simulink model "linear_model"  (Simulink 8.0)
settings: Solver=ode45  StartTime=0.0  StopTime=0.01  FixedStep=0.0001  RelTol=1e-3
settings Model: Creator=T-3000  LastModifiedBy=T-3000  BufferReuse=off
settings DataIOCC: SignalLoggingSaveFormat=ModelDataLogs  SignalLoggingName=sigsOut
settings OptimizationCC: InlineInvariantSignals=on  OptimizeBlockIOStorage=off  BufferReuse=off  ExpressionFolding=off  LocalBlockOutputs=off
settings DebuggingCC: SaveWithParameterizedLinksMsg=none  SignalResolutionControl=TryResolveAllWithWarning  SolverPrmCheckMsg=none  MultiTaskDSMMsg=warning  MultiTaskCondExecSysMsg=none  StrictBusMsg=None
settings HardwareCC: TargetUnknown=on
settings RTWCC: IncludeERTFirstTime=on
settings GRTTargetCC: CombineOutputUpdateFcns=off  GRTInterface=on

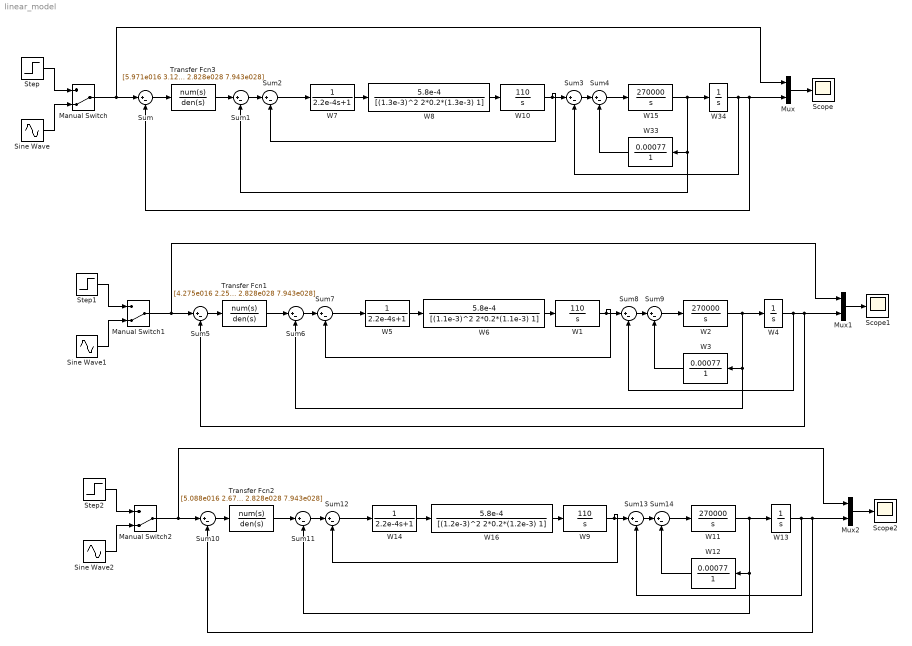
== system linear_model ==
  Manual Switch : ManualSwitch  CurrentSetting=0
  Manual Switch1 : ManualSwitch  CurrentSetting=0
  Manual Switch2 : ManualSwitch  CurrentSetting=0
  Mux : Mux  Inputs=2
  Mux1 : Mux  Inputs=2
  Mux2 : Mux  Inputs=2
  Scope : Scope
      settings: TimeRange=5  YMin=0  YMax=1.2
  Scope1 : Scope
      settings: TimeRange=5  YMin=0  YMax=1
  Scope2 : Scope
      settings: TimeRange=5  YMin=0  YMax=1  SaveName=ScopeData2
  Sine Wave : Sin  Frequency=1200  SampleTime=0
  Sine Wave1 : Sin  Frequency=1200  SampleTime=0
  Sine Wave2 : Sin  Frequency=1200  SampleTime=0
  Step : Step  Time=0  SampleTime=0
  Step1 : Step  Time=0  SampleTime=0
  Step2 : Step  Time=0  SampleTime=0
  Sum{,1..14} (15 alike) : Sum  Inputs=|+-  SaturateOnIntegerOverflow=on
  Transfer Fcn1 : TransferFcn  Numerator=[4.275e016 2.258e020 1.99e023 2.742e026 1.061e029 6.01e031 7.477e033 9.532e032]  Denominator=[1 1.539e006 8.565e011 2.152e017 2.439e022 1.001e027 2.828e028 7.943e028]
  Transfer Fcn2 : TransferFcn  Numerator=[5.088e016 2.672e020 2.225e023 2.902e026 1.101e029 6.04e031 7.477e033 9.532e032]  Denominator=[1 1.539e006 8.565e011 2.152e017 2.439e022 1.001e027 2.828e028 7.943e028]
  Transfer Fcn3 : TransferFcn  Numerator=[5.971e016 3.121e020 2.475e023 3.073e026 1.143e029 6.07e031 7.477e033 9.532e032]  Denominator=[1 1.539e006 8.565e011 2.152e017 2.439e022 1.001e027 2.828e028 7.943e028]
  W1 : TransferFcn  Numerator=[110]  Denominator=[1 0]
  W10 : TransferFcn  Numerator=[110]  Denominator=[1 0]
  W11 : TransferFcn  Numerator=[270000]  Denominator=[1 0]
  W12 : TransferFcn  Numerator=[0.00077]  Denominator=[1]
  W13 : TransferFcn  Denominator=[1 0]
  W14 : TransferFcn  Denominator=[2.2e-4 1]
  W15 : TransferFcn  Numerator=[270000]  Denominator=[1 0]
  W16 : TransferFcn  Numerator=[5.8e-4]  Denominator=[(1.2e-3)^2 2*0.2*(1.2e-3) 1]
  W2 : TransferFcn  Numerator=[270000]  Denominator=[1 0]
  W3 : TransferFcn  Numerator=[0.00077]  Denominator=[1]
  W33 : TransferFcn  Numerator=[0.00077]  Denominator=[1]
  W34 : TransferFcn  Denominator=[1 0]
  W4 : TransferFcn  Denominator=[1 0]
  W5 : TransferFcn  Denominator=[2.2e-4 1]
  W6 : TransferFcn  Numerator=[5.8e-4]  Denominator=[(1.1e-3)^2 2*0.2*(1.1e-3) 1]
  W7 : TransferFcn  Denominator=[2.2e-4 1]
  W8 : TransferFcn  Numerator=[5.8e-4]  Denominator=[(1.3e-3)^2 2*0.2*(1.3e-3) 1]
  W9 : TransferFcn  Numerator=[110]  Denominator=[1 0]
  wires:
  Sum2/1 -> W7/1
  W7/1 -> W8/1
  W8/1 -> W10/1
  W10/1 -> Sum3/1, Sum2/2
  Sum3/1 -> Sum4/1
  Sum4/1 -> W15/1
  W15/1 -> Sum1/2, W33/1, W34/1
  Step/1 -> Manual Switch/1
  Sine Wave/1 -> Manual Switch/2
  Mux/1 -> Scope/1
  Manual Switch/1 -> Mux/1, Sum/1
  Sum1/1 -> Sum2/1
  W34/1 -> Sum3/2, Sum/2, Mux/2
  W33/1 -> Sum4/2
  Sum7/1 -> W5/1
  W5/1 -> W6/1
  W6/1 -> W1/1
  W1/1 -> Sum8/1, Sum7/2
  Sum8/1 -> Sum9/1
  Sum9/1 -> W2/1
  W2/1 -> Sum6/2, W3/1, W4/1
  Step1/1 -> Manual Switch1/1
  Sine Wave1/1 -> Manual Switch1/2
  Mux1/1 -> Scope1/1
  Manual Switch1/1 -> Mux1/1, Sum5/1
  Sum6/1 -> Sum7/1
  Sum5/1 -> Transfer Fcn1/1
  W4/1 -> Sum8/2, Sum5/2, Mux1/2
  W3/1 -> Sum9/2
  Transfer Fcn1/1 -> Sum6/1
  Sum12/1 -> W14/1
  W14/1 -> W16/1
  W16/1 -> W9/1
  W9/1 -> Sum13/1, Sum12/2
  Sum13/1 -> Sum14/1
  Sum14/1 -> W11/1
  W11/1 -> Sum11/2, W12/1, W13/1
  Step2/1 -> Manual Switch2/1
  Sine Wave2/1 -> Manual Switch2/2
  Mux2/1 -> Scope2/1
  Manual Switch2/1 -> Mux2/1, Sum10/1
  Sum11/1 -> Sum12/1
  Sum10/1 -> Transfer Fcn2/1
  W13/1 -> Sum13/2, Sum10/2, Mux2/2
  W12/1 -> Sum14/2
  Transfer Fcn2/1 -> Sum11/1
  Sum/1 -> Transfer Fcn3/1
  Transfer Fcn3/1 -> Sum1/1
